simulink model "test_observer_2018B"  (R2018b)
settings: Solver=VariableStepAuto  StartTime=0.0  StopTime=4  RelTol=1e-3
libraries: simulink x2
settings Model: Creator=Alex  LastModifiedBy=timof
settings DataIOCC: ReturnWorkspaceOutputs=on
settings DebuggingCC: UnconnectedInputMsg=none  UnconnectedOutputMsg=none  UnconnectedLineMsg=none  SFMachineParentedDataDiag=error

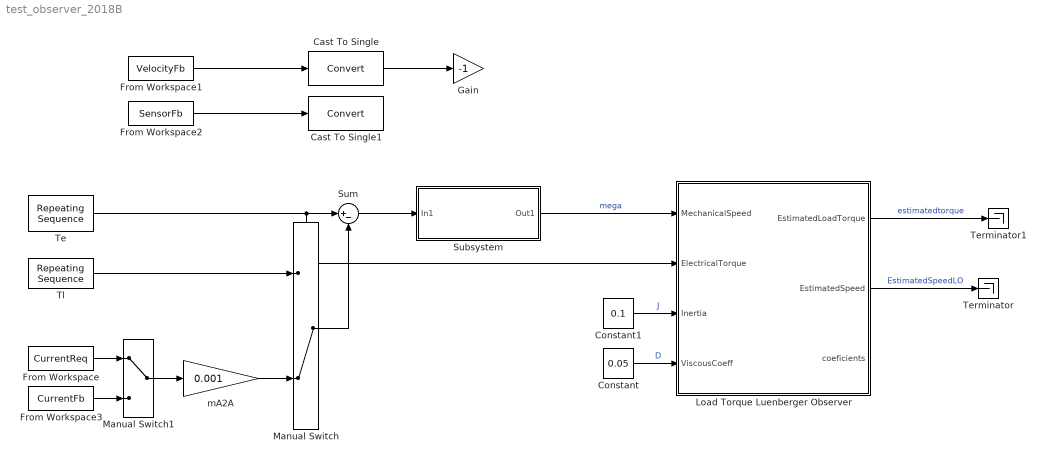
== system test_observer_2018B ==
  Cast To Single : DataTypeConversion
  Cast To Single1 : DataTypeConversion
  Constant : Constant  Value=0.05
  Constant1 : Constant  Value=0.1
  From Workspace : FromWorkspace  VariableName=CurrentReq  SampleTime=0
  From Workspace1 : FromWorkspace  VariableName=VelocityFb  SampleTime=0
  From Workspace2 : FromWorkspace  VariableName=SensorFb  SampleTime=0
  From Workspace3 : FromWorkspace  VariableName=CurrentFb  SampleTime=0
  Gain : Gain  Gain=-1
  Load Torque Luenberger Observer : MATLAB Function  TreatAsAtomicUnit=on  SystemSampleTime=5e-3
  Manual Switch : ManualSwitch  CurrentSetting=0
  Manual Switch1 : ManualSwitch
  Subsystem : Subsystem
  Sum : Sum  Inputs=|+-
  Te : simulink/Sources/Repeating Sequence  rep_seq_t=[0 2 2.001 3 3.001 5 5.001]  rep_seq_y=[5 5 0 0 -5 -5 0]*0
  Terminator : Terminator
  Terminator1 : Terminator
  Tl : simulink/Sources/Repeating Sequence  rep_seq_t=[0 1 1.0001 2.5 2.50001 4 4.0001 4.5 4.50001]  rep_seq_y="[0 0 2  2 0 0 -2 -2 0]"
  mA2A : Gain  Gain=0.001
  wires:
  Constant1/1 -> Load Torque Luenberger Observer/3(Inertia)  "J"
  Constant/1 -> Load Torque Luenberger Observer/4(ViscousCoeff)  "D"
  Subsystem/1(Out1) -> Load Torque Luenberger Observer/1(MechanicalSpeed)  "mega"
  Te/1 -> Load Torque Luenberger Observer/2(ElectricalTorque), Sum/1
  Tl/1 -> Manual Switch/1
  Load Torque Luenberger Observer/2(EstimatedSpeed) -> Terminator/1  "EstimatedSpeedLO"
  Load Torque Luenberger Observer/1(EstimatedLoadTorque) -> Terminator1/1  "estimatedtorque"
  From Workspace/1 -> Manual Switch1/1
  Manual Switch/1 -> Sum/2
  mA2A/1 -> Manual Switch/2
  Sum/1 -> Subsystem/1(In1)
  From Workspace1/1 -> Cast To Single/1
  Cast To Single/1 -> Gain/1
  From Workspace2/1 -> Cast To Single1/1
  From Workspace3/1 -> Manual Switch1/2
  Manual Switch1/1 -> mA2A/1

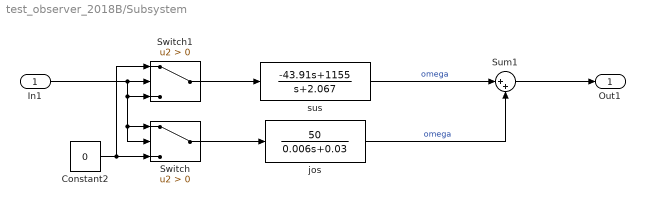
== system test_observer_2018B/Subsystem ==
  In1 : Inport
  Constant2 : Constant  Value=0  SampleTime=2
  Sum1 : Sum  Inputs=|++
  Switch : Switch  Criteria=u2 > Threshold
  Switch1 : Switch  Criteria=u2 > Threshold
  jos : TransferFcn  Numerator=[50]  Denominator=[0.006 0.03]
  sus : TransferFcn  Numerator=[-43.91, 1155]  Denominator=[1,2.067]
  Out1 : Outport
  wires:
  Sum1/1 -> Out1/1
  In1/1 -> Switch/2, Switch/1, Switch1/3, Switch1/2
  sus/1 -> Sum1/1  "omega"
  Switch/1 -> jos/1
  Switch1/1 -> sus/1
  Constant2/1 -> Switch1/1, Switch/3
  jos/1 -> Sum1/2  "omega"

== matlab function test_observer_2018B/Load Torque Luenberger Observer ==
  data: MechanicalSpeed input; ElectricalTorque input; Inertia input; ViscousCoeff input; EstimatedLoadTorque output; EstimatedSpeed output; coeficients output
function [EstimatedLoadTorque,EstimatedSpeed,coeficients] = LoadLO(MechanicalSpeed, ElectricalTorque, Inertia,ViscousCoeff)

coder.extrinsic('place');
persistent x;
persistent Phi;
persistent Gamma;
persistent L;

SamplingTime = single(5e-3);
if(isempty(x))
    x = single([0; 0]);
    A = single([-ViscousCoeff/Inertia -1/Inertia; 0 0]);
    B = single([1/Inertia; 0]);
    C = [1 0];
    Phi = single(eye(2)+A*SamplingTime+1/2*(A*SamplingTime)*(A*SamplingTime));
    Gamma = single((eye(2)+1/2*SamplingTime * A+1/6*(A*SamplingTime)*(A*SamplingTime))*SamplingTime*B);
    
    des_ttime = 0.5*100e-3;
    cpole1 = - 4/des_ttime;
    cpole2 = - 4/des_ttime/2;
    dpoles = exp([cpole1;cpole2]*SamplingTime);
    L = single([ 0 ; 0]);
    coeficients = single([ 0 ; 0]);
    
    L = place(Phi',C',dpoles')';
    
    %L = single([0.1151; -0.0024]); %MKC1
%     L = single([0.1151; -0.00341]); %MKC2
end

% Run state-space equation
x = Phi * x + Gamma * ElectricalTorque + L *(MechanicalSpeed-x(1));
EstimatedSpeed = x(1);
EstimatedLoadTorque = x(2);
coeficients = L;
end
